simulink model "Lyapunov_Control"  (R2015b)
settings: Solver=ode8  StartTime=5  StopTime=26  FixedStep=0.1  RelTol=1e-3
values from neighbouring files (symbols this model uses):
  Ktheta = 10    [init.m]
  Kx = 10    [init.m]
  Ky = 10    [init.m]
  L = 0.13    [init.m]
  r = 0.1    [init.m]
  R = 2    [init.m]
  Theta0 = pi    (= 3.14159265359)    [init.m]
  wd = 0.5    [init.m]
  X0 = 2.3    [init.m]
  Y0 = 0    [init.m]
undefined symbols (not defined in the file): alpha
libraries: simulink x2
settings Model: Creator=GANESH  LastModifiedBy=GANESH
settings SolverCC: AlgebraicLoopSolver=LineSearch

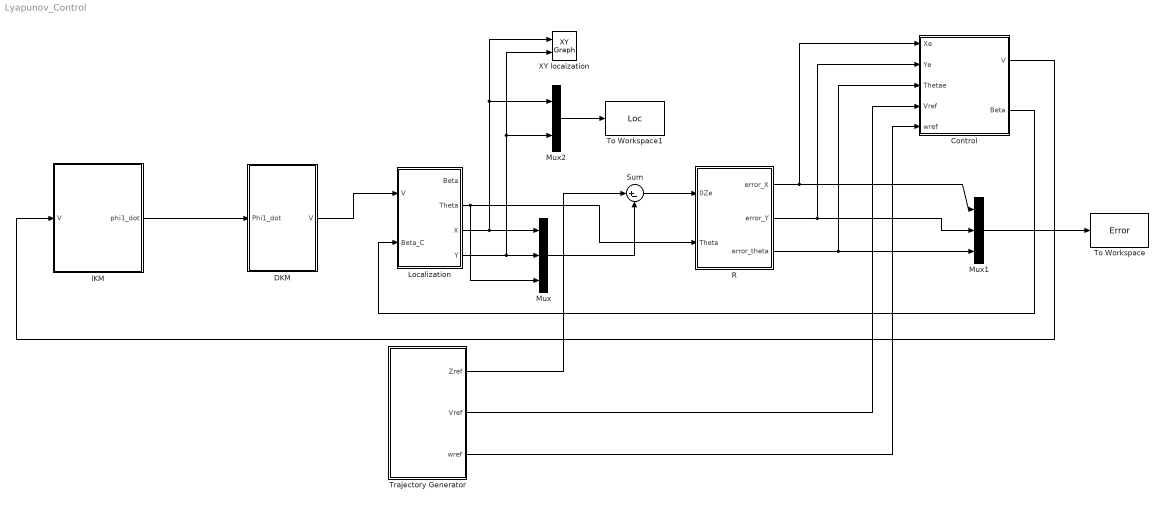
== system Lyapunov_Control ==
  Control : Subsystem
  DKM : Subsystem  mask{r=r}
      mask prompts: r "Radius of the Wheel"
  IKM : Subsystem  mask{r=(1+alpha)*r}
      mask prompts: r "Radius of the Wheel"
  Localization : Subsystem  mask{L=L}
      mask prompts: L "Half of WheelBase"
  Mux : Mux  Inputs=3
  Mux1 : Mux  Inputs=3
  Mux2 : Mux  Inputs=2
  R : Subsystem
  Sum : Sum  Inputs=|+-
  To Workspace : ToWorkspace  VariableName=Error  SaveFormat=Timeseries  SampleTime=-1
  To Workspace1 : ToWorkspace  VariableName=Loc  SaveFormat=Timeseries  SampleTime=-1
  Trajectory Generator : Subsystem  mask{R=R, wd=wd}
      mask prompts: R "Radius of Circular Trajectory"; wd "Desired Angular Velocity"
  XY locaization : simulink/Sinks/XY Graph  xmin=-5  xmax=5  ymin=-5  ymax=5  st=-1
  wires:
  IKM/1(phi1_dot) -> DKM/1(Phi1_dot)
  R/1(error_X) -> Control/1(Xe), Mux1/1
  R/2(error_Y) -> Control/2(Ye), Mux1/2
  R/3(error_theta) -> Control/3(Thetae), Mux1/3
  Trajectory Generator/2(Vref) -> Control/4("Vref ")
  Trajectory Generator/3(wref) -> Control/5(wref)
  Trajectory Generator/1(Zref) -> Sum/1
  Mux/1 -> Sum/2
  Sum/1 -> R/1(0Ze)
  DKM/1(V) -> Localization/1(V)
  Localization/3(X) -> XY locaization/1, Mux2/1, Mux/1
  Localization/4(Y) -> XY locaization/2, Mux2/2, Mux/2
  Localization/2(Theta) -> R/2(Theta), Mux/3
  Control/1(V) -> IKM/1(V)
  Control/2(Beta) -> Localization/2(Beta_C)
  Mux1/1 -> To Workspace/1
  Mux2/1 -> To Workspace1/1

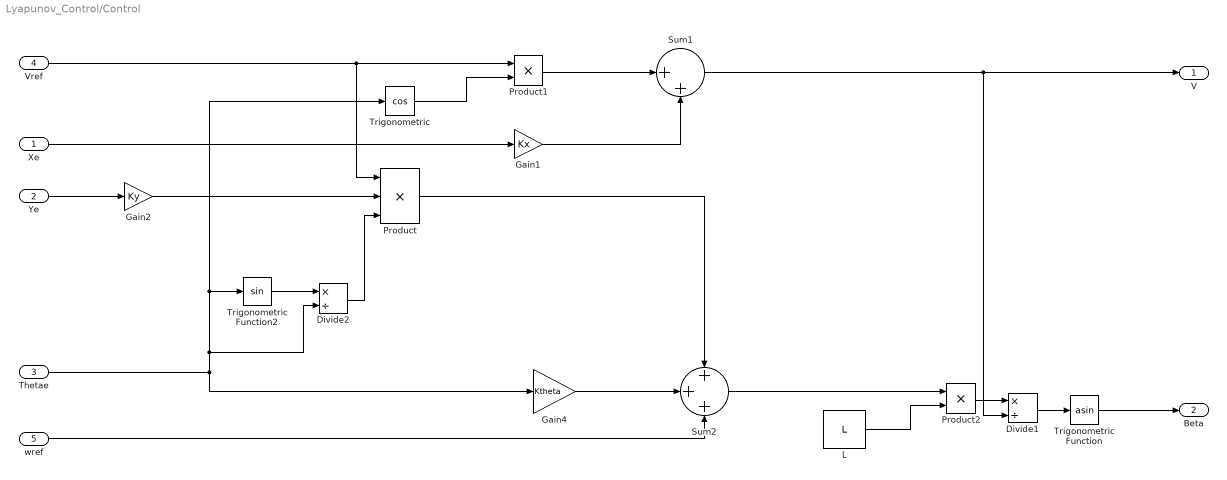
== system Lyapunov_Control/Control ==
  Xe : Inport
  Ye : Inport  Port=2
  Thetae : Inport  Port=3
  "Vref " : Inport  Port=4
  wref : Inport  Port=5
  Divide1 : Product  Inputs=*/
  Divide2 : Product  Inputs=*/
  Gain1 : Gain  Gain=Kx
  Gain2 : Gain  Gain=Ky
  Gain4 : Gain  Gain=Ktheta
  L : Constant  Value=L
  Product : Product  Inputs=3
  Product1 : Product
  Product2 : Product
  Sum1 : Sum  Inputs=|++
  Sum2 : Sum  Inputs=+++
  "Trigonometric " : Trigonometry  Operator=cos
  Trigonometric Function : Trigonometry  Operator=asin
  Trigonometric Function2 : Trigonometry
  V : Outport
  Beta : Outport  Port=2
  wires:
  "Trigonometric "/1 -> Product1/2
  Xe/1 -> Gain1/1
  Thetae/1 -> Gain4/1, "Trigonometric "/1, Trigonometric Function2/1, Divide2/2
  Product/1 -> Sum2/1
  Gain4/1 -> Sum2/2
  Product1/1 -> Sum1/1
  Gain1/1 -> Sum1/2
  "Vref "/1 -> Product/1, Product1/1
  wref/1 -> Sum2/3
  Trigonometric Function2/1 -> Divide2/1
  Divide2/1 -> Product/3
  Ye/1 -> Gain2/1
  Gain2/1 -> Product/2
  Trigonometric Function/1 -> Beta/1
  L/1 -> Product2/2
  Sum1/1 -> Divide1/2, V/1
  Sum2/1 -> Product2/1
  Product2/1 -> Divide1/1
  Divide1/1 -> Trigonometric Function/1

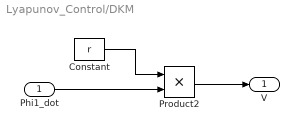
== system Lyapunov_Control/DKM ==
  Phi1_dot : Inport
  Constant : Constant  Value=r
  Product2 : Product
  V : Outport
  wires:
  Phi1_dot/1 -> Product2/2
  Constant/1 -> Product2/1
  Product2/1 -> V/1

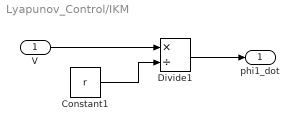
== system Lyapunov_Control/IKM ==
  V : Inport
  Constant1 : Constant  Value=r
  Divide1 : Product  Inputs=*/
  phi1_dot : Outport
  wires:
  V/1 -> Divide1/1
  Constant1/1 -> Divide1/2
  Divide1/1 -> phi1_dot/1

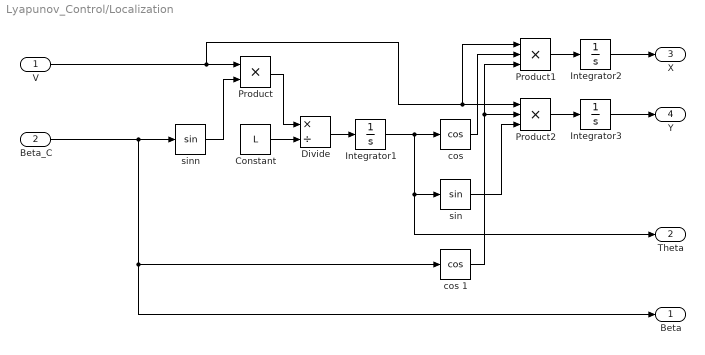
== system Lyapunov_Control/Localization ==
  V : Inport
  Beta_C : Inport  Port=2
  Constant : Constant  Value=L
  Divide : Product  Inputs=*/
  Integrator1 : Integrator  InitialCondition=Theta0
  Integrator2 : Integrator  InitialCondition=X0
  Integrator3 : Integrator  InitialCondition=Y0
  Product : Product
  Product1 : Product  Inputs=3
  Product2 : Product  Inputs=3
  "cos " : Trigonometry  Operator=cos
  cos 1 : Trigonometry  Operator=cos
  sin : Trigonometry
  sinn : Trigonometry
  Beta : Outport
  Theta : Outport  Port=2
  X : Outport  Port=3
  Y : Outport  Port=4
  wires:
  Integrator1/1 -> Theta/1, sin/1, "cos "/1
  Product2/1 -> Integrator3/1
  Integrator3/1 -> Y/1
  V/1 -> Product1/1, Product2/1, Product/1
  Product/1 -> Divide/1
  Product1/1 -> Integrator2/1
  Integrator2/1 -> X/1
  Divide/1 -> Integrator1/1
  Beta_C/1 -> Beta/1, cos 1/1, sinn/1
  sinn/1 -> Product/2
  Constant/1 -> Divide/2
  cos 1/1 -> Product1/3, Product2/2
  "cos "/1 -> Product1/2
  sin/1 -> Product2/3

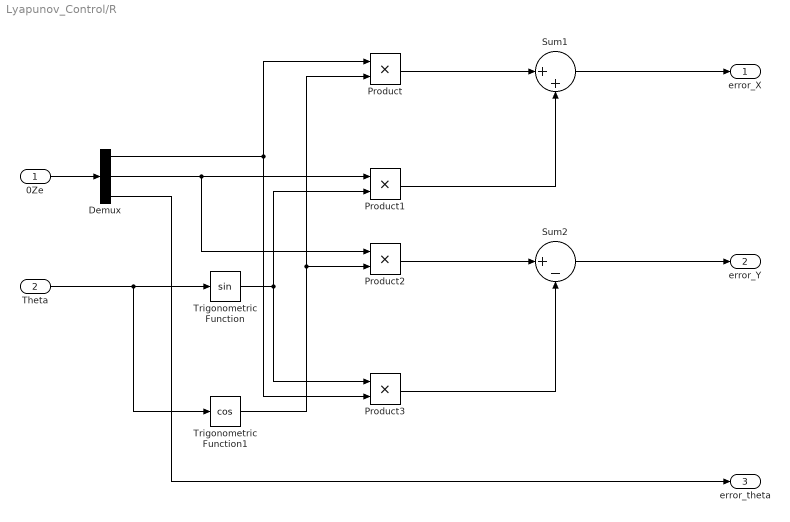
== system Lyapunov_Control/R ==
  0Ze : Inport
  Theta : Inport  Port=2
  Demux : Demux  Outputs=3
  Product{,1..3} (4 alike) : Product
  Sum1 : Sum  Inputs=|++
  Sum2 : Sum  Inputs=|+-
  Trigonometric Function : Trigonometry
  Trigonometric Function1 : Trigonometry  Operator=cos
  error_X : Outport
  error_Y : Outport  Port=2
  error_theta : Outport  Port=3
  wires:
  Theta/1 -> Trigonometric Function/1, Trigonometric Function1/1
  Sum1/1 -> error_X/1
  Sum2/1 -> error_Y/1
  Demux/1 -> Product3/2, Product/1
  Trigonometric Function1/1 -> Product2/2, Product/2
  Product/1 -> Sum1/1
  Demux/2 -> Product1/1, Product2/1
  Trigonometric Function/1 -> Product3/1, Product1/2
  Product1/1 -> Sum1/2
  Product2/1 -> Sum2/1
  Product3/1 -> Sum2/2
  Demux/3 -> error_theta/1
  0Ze/1 -> Demux/1

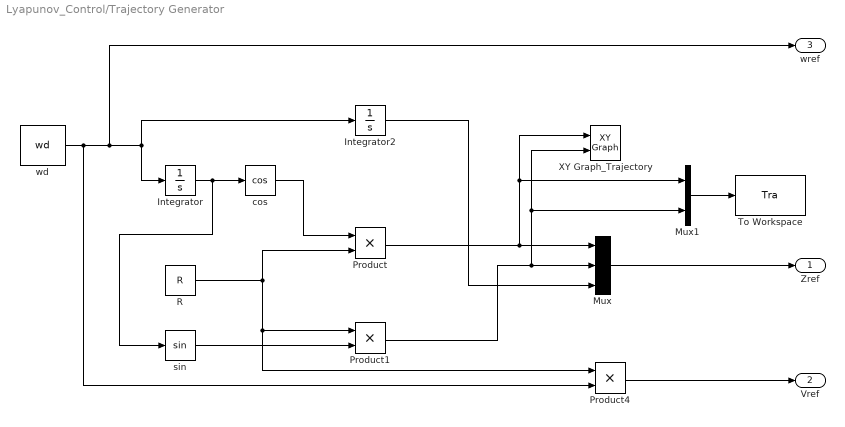
== system Lyapunov_Control/Trajectory Generator ==
  Integrator : Integrator
  Integrator2 : Integrator  InitialCondition=pi/2
  Mux : Mux  Inputs=3
  Mux1 : Mux  Inputs=2
  Product : Product
  Product1 : Product
  Product4 : Product
  R : Constant  Value=R
  To Workspace : ToWorkspace  VariableName=Tra  SaveFormat=Timeseries  SampleTime=-1
  XY Graph_Trajectory : simulink/Sinks/XY Graph  xmin=-5  xmax=5  ymin=-5  ymax=5  st=-1
  cos : Trigonometry  Operator=cos
  sin : Trigonometry
  wd : Constant  Value=wd
  Zref : Outport
  Vref : Outport  Port=2
  wref : Outport  Port=3
  wires:
  R/1 -> Product4/1, Product1/1, Product/2
  Product1/1 -> XY Graph_Trajectory/2, Mux1/2, Mux/2
  Product/1 -> XY Graph_Trajectory/1, Mux1/1, Mux/1
  wd/1 -> Product4/2, wref/1, Integrator2/1, Integrator/1
  Integrator/1 -> sin/1, cos/1
  Product4/1 -> Vref/1
  cos/1 -> Product/1
  sin/1 -> Product1/2
  Integrator2/1 -> Mux/3
  Mux/1 -> Zref/1
  Mux1/1 -> To Workspace/1
